simulink model "model"  (R2019b)
settings: Solver=VariableStepAuto  StartTime=0.0  StopTime=60  RelTol=1e-3
model workspace: external: MATLAB File C:\Users\thoma\OneDrive\Documents\University Work\Fourth Year\Semester 1 2022\Thesis\MATLAB Code\Thesis\2D 3DOF Model\twoD_test.m (data not in the file)
values from neighbouring files (symbols this model uses):
  A = [I_alpha, (I_beta + b(c-a)*S_beta), S_alpha ... (first row only)    [Theodoresen_Model.m]
  C = CkCalculation(k)    [Aerodynamic_Forces_Calculation.m]    (also in CkCalculation.m = complex(F, G); Theodoresen_Model.m = C_k_Laplace(v, b, 0.01))
undefined symbols (not defined in the file or in its folder): x0
settings Model: Creator=thoma  LastModifiedBy=thoma

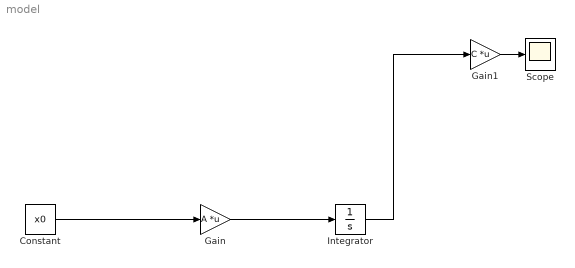
== system model ==
  Constant : Constant  Value=x0
  Gain : Gain  Gain=A  Multiplication=Matrix(K*u)
  Gain1 : Gain  Gain=C  Multiplication=Matrix(K*u)
  Integrator : Integrator
  Scope : Scope
  wires:
  Gain/1 -> Integrator/1
  Integrator/1 -> Gain1/1
  Constant/1 -> Gain/1
  Gain1/1 -> Scope/1
